simulink model "Task1"  (R2020b)
settings: Solver=ode4  StartTime=0.0  StopTime=10  FixedStep=1e-3  RelTol=1e-3
InitFcn:
  | acm_init
values from neighbouring files (symbols this model uses):
  alpha = 5    [acm_init.m]
  fd1 = 5.3    [acm_init.m]
  fd2 = 1.1    [acm_init.m]
  k = [50;50]    [acm_init.m]
  p1 = 3.473    [acm_init.m]
  p2 = 0.196    [acm_init.m]
  p3 = 0.242    [acm_init.m]
settings Model: Creator=Tenghu  LastModifiedBy=jsol
settings SolverCC: ZeroCrossControl=EnableAll  AlgebraicLoopSolver=LineSearch
settings DataIOCC: SaveFormat=StructureWithTime
settings OptimizationCC: BlockReduction=off  BooleanDataType=off  LifeSpan=inf
settings DebuggingCC: SaveWithParameterizedLinksMsg=none  UnderspecifiedInitializationDetection=Classic  MergeDetectMultiDrivingBlocksExec=none  SignalResolutionControl=TryResolveAllWithWarning  AllowSymbolicDim=off  SFUnexpectedBacktrackingDiag=warning  SFNoUnconditionalDefaultTransitionDiag=warning  SFExecutionAtInitializationDiag=none  ArithmeticOperatorsInVariantConditions=warning
settings HardwareCC: ProdBitPerPointer=32  ProdBitPerSizeT=32  ProdBitPerPtrDiffT=32  ProdLargestAtomicFloat=None  ProdIntDivRoundTo=Undefined  ProdEndianess=Unspecified  ProdWordSize=32  ProdHWDeviceType=32-bit Generic  TargetBitPerPointer=64  TargetBitPerSizeT=64  TargetBitPerPtrDiffT=64  TargetLongLongMode=on  TargetIntDivRoundTo=Zero  TargetEndianess=LittleEndian  TargetWordSize=64  TargetHWDeviceType=MATLAB Host  ProdEqTarget=off
settings ModelReferenceCC: PropagateSignalLabelsOutOfModel=off
settings SFSimCC: SimUseLocalCustomCode=off  CustomCodeUndefinedFunction=UseInterfaceOnly
settings RTWCC: RTWUseLocalCustomCode=off
settings CodeAppCC: StateflowObjectComments=on
settings GRTTargetCC: TargetLangStandard=C89/C90 (ANSI)
settings ConfigComp: CovMetricSettings=dw  CovSaveCumulativeToWorkspaceVar=on  CovSaveSingleToWorkspaceVar=on  CovExternalEMLEnable=off  CovSFcnEnable=off

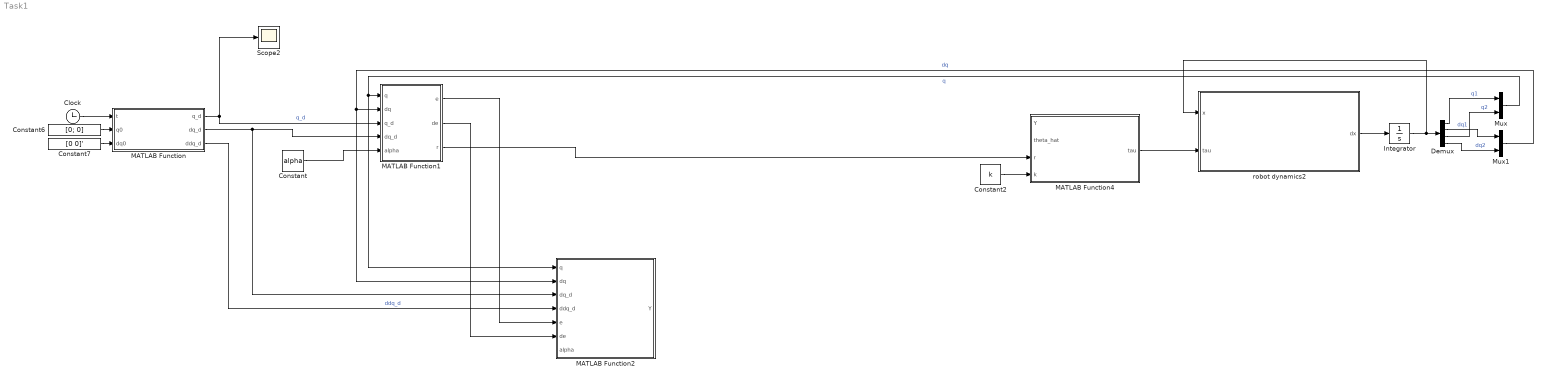
== system Task1 ==
  Clock : Clock
  Constant : Constant  Value=alpha
  Constant2 : Constant  Value=k
  Constant6 : Constant  Value=[0; 0]
  Constant7 : Constant  Value=[0 0]'
  Demux : Demux
  Integrator : Integrator
  MATLAB Function : MATLAB Function  TreatAsAtomicUnit=on
  MATLAB Function1 : MATLAB Function  TreatAsAtomicUnit=on
  MATLAB Function2 : MATLAB Function  TreatAsAtomicUnit=on
  MATLAB Function4 : MATLAB Function  TreatAsAtomicUnit=on
  Mux : Mux  Inputs=2
  Mux1 : Mux  Inputs=2
  Scope2 : Scope
  robot dynamics2 : MATLAB Function  TreatAsAtomicUnit=on
  wires:
  Clock/1 -> MATLAB Function/1(t)
  Constant7/1 -> MATLAB Function/3(dq0)
  Constant6/1 -> MATLAB Function/2(q0)
  MATLAB Function/1(q_d) -> Scope2/1, MATLAB Function1/3(q_d)  "q_d"
  robot dynamics2/1(dx) -> Integrator/1
  Integrator/1 -> Demux/1, robot dynamics2/1(x)
  MATLAB Function4/1(tau) -> robot dynamics2/2(tau)
  Constant2/1 -> MATLAB Function4/4(k)
  Demux/1 -> Mux/1  "q1"
  Demux/3 -> Mux/2  "q2"
  Demux/4 -> Mux1/2  "dq2"
  MATLAB Function/2(dq_d) -> MATLAB Function2/3(dq_d), MATLAB Function1/4(dq_d)
  Demux/2 -> Mux1/1  "dq1"
  Mux/1 -> MATLAB Function2/1(q), MATLAB Function1/1(q)  "q"
  Mux1/1 -> MATLAB Function2/2(dq), MATLAB Function1/2(dq)  "dq"
  Constant/1 -> MATLAB Function1/5(alpha)
  MATLAB Function1/3(r) -> MATLAB Function4/3(r)
  MATLAB Function/3(ddq_d) -> MATLAB Function2/4(ddq_d)  "ddq_d"
  MATLAB Function1/1(e) -> MATLAB Function2/5(e)
  MATLAB Function1/2(de) -> MATLAB Function2/6(de)

== matlab function Task1/MATLAB Function2 ==
  data: q input; dq input; Y output; dq_d input; ddq_d input; e input; de input; alpha input
function Y = regressor_matrix(q,dq,dq_d,ddq_d,e,de,alpha)

% Intermediate terms
sigma1 = ddq_d + alpha * de;
sigma2 = dq_d + alpha * e;
sigma3 = dq;  

% Trigonometric terms
c2 = cos(q(2));
s2 = sin(q(2));

% Initialize regressor matrix
Y = zeros(2, 5);

% Row 1
Y(1,1) = sigma1(1);
Y(1,2) = sigma1(2);
Y(1,3) = 2 * c2 * sigma1(1) + c2 * sigma1(2)-s2 * dq(2) * sigma2(1) - s2 * (dq(1) + dq(2)) * sigma2(2);
Y(1,4) = sigma3(1);
Y(1,5) = 0;

% Row 2
Y(2,1) = 0;
Y(2,2) = sigma1(1) + sigma1(2);
Y(2,3) = c2 * sigma1(1) + s2 * dq(1) * sigma2(1);
Y(2,4) = 0;
Y(2,5) = sigma3(2);

== matlab function Task1/MATLAB Function1 ==
  data: q input; dq input; e output; q_d input; dq_d input; alpha input; de output; r output
function [e, de, r] = error(q,dq,q_d,dq_d,alpha)


e = q_d-q;
de = dq_d-dq;

r = de + alpha*e;

== matlab function Task1/MATLAB Function4 ==
  data: Y input; theta_hat input; tau output; r input; k input
function tau = controller_law(Y,theta_hat,r,k)

tau = k*r + Y*theta_hat;

== matlab function Task1/MATLAB Function ==
  data: t input; q_d output; q0 input; dq0 input; dq_d output; ddq_d output
function [q_d, dq_d, ddq_d] = desired_traj(t,q0,dq0)
   
    q_d   = [sin(3*t);2*cos(t)] + dq0*t + q0;
    dq_d  = [3*cos(3*t); -2*sin(t)] + dq0;
    ddq_d = [-9*cos(3*t); -2*cos(t)];
end

== matlab function Task1/robot dynamics2 ==
  data: x input; dx output; tau input; p1 parameter; p2 parameter; p3 parameter; fd1 parameter; fd2 parameter
% *************************************************************************
%                        2-Link Manipulator Dynamics                      *
% *************************************************************************

function dx = fcn_twoLinkDynamics(x, tau, p1, p2, p3, fd1, fd2)
    q1  = x(1);
    dq1 = x(2);
    q2  = x(3);
    dq2 = x(4);
    
    M      = zeros(2,2);
    M(1,1) = p1 + 2*p3*cos(q2);
    M(1,2) = p2 + p3*cos(q2);
    M(2,1) = p2 + p3*cos(q2);
    M(2,2) = p2;

    C      = zeros(2,2);
    C(1,1) = -p3*sin(q2)*dq2;
    C(1,2) = -p3*sin(q2)*(dq1+dq2);
    C(2,1) = p3*sin(q2)*dq1;
    C(2,2) = 0;

    Fd     = diag([fd1 fd2]);

    % The system without bounded disturbances =============================
    ddq = M\(tau - C*[dq1;dq2] - Fd*[dq1;dq2]);
    dx  = [dq1; ddq(1); dq2; ddq(2)];
end
